simulink model "AME552_HW2_P1_SimulinkModel"  (R2024b)
settings: Solver=VariableStepAuto  StartTime=0.0  StopTime=10  RelTol=1e-6
values from neighbouring files (symbols this model uses):
  A = 1    [AME552_HW2_P1.m]    (also in AME552_HW2_P1_Simulink.m)
  D = 1    [AME552_HW2_P1.m]    (also in AME552_HW2_P1_Simulink.m)
  de0 = de0_space(j)    [AME552_HW2_P1_Simulink.m]
  e0 = e0_space(i)    [AME552_HW2_P1_Simulink.m]
  I = 1    [AME552_HW2_P1.m]    (also in AME552_HW2_P1_Simulink.m)
  tau = 1    [AME552_HW2_P1.m]    (also in AME552_HW2_P1_Simulink.m)
libraries: simulink x1
settings Model: Creator=lewis  LastModifiedBy=lewis

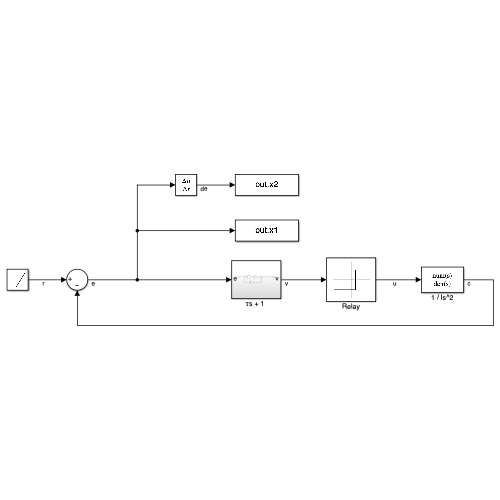
[thumbnail: Simulink's stored preview of the top-level diagram]
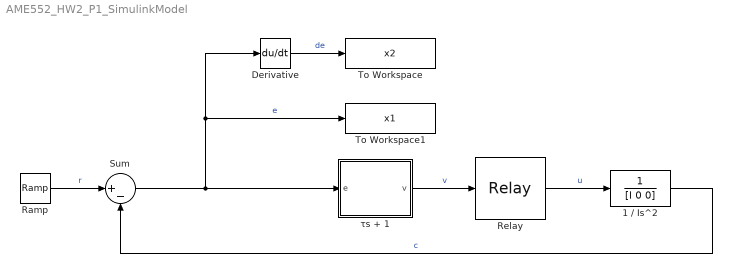
== system AME552_HW2_P1_SimulinkModel ==
  1 / Is^2 : TransferFcn  Denominator=[I 0 0]
  Derivative : Derivative
  Ramp : simulink/Sources/Ramp  slope=de0  start=0  InitialOutput=e0
  Relay : Relay  OnSwitchValue=D  OffSwitchValue=-D  OnOutputValue=A  OffOutputValue=-A
  Sum : Sum  Inputs=|+-
  To Workspace : ToWorkspace  VariableName=x2  SaveFormat=Timeseries  SampleTime=-1
  To Workspace1 : ToWorkspace  VariableName=x1  SaveFormat=Timeseries  SampleTime=-1
  "τs + 1 " : Subsystem
  wires:
  Relay/1 -> 1 / Is^2/1  "u"
  Sum/1 -> "τs + 1 "/1(e), To Workspace1/1, Derivative/1  "e"
  "τs + 1 "/1(v) -> Relay/1  "v"
  Derivative/1 -> To Workspace/1  "de"
  1 / Is^2/1 -> Sum/2  "c"
  Ramp/1 -> Sum/1  "r"

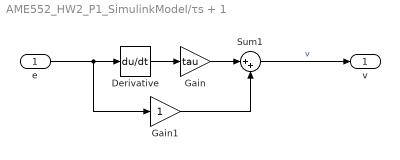
== system AME552_HW2_P1_SimulinkModel/τs + 1  ==
  e : Inport
  Derivative : Derivative
  Gain : Gain  Gain=tau
  Gain1 : Gain
  Sum1 : Sum  Inputs=|++
  v : Outport
  wires:
  Gain1/1 -> Sum1/2
  Gain/1 -> Sum1/1
  Derivative/1 -> Gain/1
  Sum1/1 -> v/1  "v"
  e/1 -> Gain1/1, Derivative/1
